simulink model "Test_inverse_kinematics"  (R2017a)
settings: Solver=VariableStepAuto  StartTime=0.0  StopTime=T  RelTol=1e-3
InitFcn:
  | KUKA_LBR_init
values from neighbouring files (symbols this model uses):
  elbowAngle = elbowAngle * pi/180    (= 0)    [KUKA_LBR_init.m]    (also in Untitled2.m)
  Kuka_LBR_param_simu = Simulink.Parameter(Kuka_LBR_param_simu)    [KUKA_LBR_init.m]
  rpyDes = rpyDes * pi/180    [KUKA_LBR_init.m]    (also in Untitled2.m)
  T = 0.5    [KUKA_LBR_init.m]
  vecGlobalConfig = [1; 1; 1]    [KUKA_LBR_init.m]    (also in Untitled2.m = [1, 1, 1])
settings Model: Creator=pc  LastModifiedBy=pc

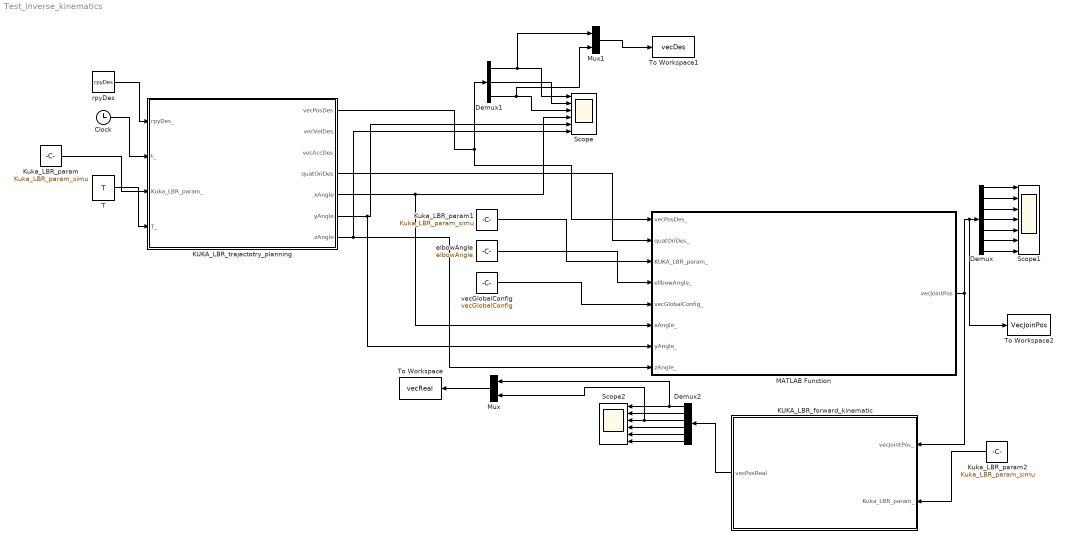
== system Test_inverse_kinematics ==
  Clock : Clock
  Demux : Demux  Outputs=7
  Demux1 : Demux  Outputs=3
  Demux2 : Demux  Outputs=6
  KUKA_LBR_forward_kinematic : MATLAB Function  TreatAsAtomicUnit=on
  KUKA_LBR_trajectotry_planning : MATLAB Function  TreatAsAtomicUnit=on
  Kuka_LBR_param : Constant  Value=Kuka_LBR_param_simu  OutDataTypeStr=Bus: Kuka_LBR_param_simu_Type
  Kuka_LBR_param1 : Constant  Value=Kuka_LBR_param_simu  OutDataTypeStr=Bus: Kuka_LBR_param_simu_Type
  Kuka_LBR_param2 : Constant  Value=Kuka_LBR_param_simu  OutDataTypeStr=Bus: Kuka_LBR_param_simu_Type
  MATLAB Function : MATLAB Function  TreatAsAtomicUnit=on
  Mux : Mux  Inputs=2
  Mux1 : Mux  Inputs=2
  Scope : Scope  NumInputPorts=6
  Scope1 : Scope  NumInputPorts=7
  Scope2 : Scope  NumInputPorts=6
  T : Constant  Value=T
  To Workspace : ToWorkspace  VariableName=vecReal  SaveFormat=Timeseries  SampleTime=-1
  To Workspace1 : ToWorkspace  VariableName=vecDes  SaveFormat=Timeseries  SampleTime=-1
  To Workspace2 : ToWorkspace  VariableName=VecJoinPos  SaveFormat=Timeseries  SampleTime=-1
  elbowAngle : Constant  Value=elbowAngle
  rpyDes : Constant  Value=rpyDes
  vecGlobalConfig : Constant  Value=vecGlobalConfig
  wires:
  Kuka_LBR_param1/1 -> MATLAB Function/3(KUKA_LBR_param_)
  rpyDes/1 -> KUKA_LBR_trajectotry_planning/1(rpyDes_)
  Clock/1 -> KUKA_LBR_trajectotry_planning/2(t_)
  Kuka_LBR_param/1 -> KUKA_LBR_trajectotry_planning/3(Kuka_LBR_param_)
  KUKA_LBR_trajectotry_planning/4(quatOriDes) -> MATLAB Function/2(quatOriDes_)
  T/1 -> KUKA_LBR_trajectotry_planning/4(T_)
  KUKA_LBR_trajectotry_planning/1(vecPosDes) -> Demux1/1, MATLAB Function/1(vecPosDes_)
  vecGlobalConfig/1 -> MATLAB Function/5(vecGlobalConfig_)
  elbowAngle/1 -> MATLAB Function/4(ellbowAngle_)
  MATLAB Function/1(vecJointPos) -> To Workspace2/1, Demux/1, KUKA_LBR_forward_kinematic/1(vecJointPos_)
  Demux/7 -> Scope1/7
  Demux/6 -> Scope1/6
  Demux/5 -> Scope1/5
  Demux/4 -> Scope1/4
  Demux/3 -> Scope1/3
  Demux/2 -> Scope1/2
  Demux/1 -> Scope1/1
  Demux1/1 -> Mux1/1, Scope/1
  Demux1/2 -> Scope/2
  Demux1/3 -> Mux1/2, Scope/3
  Demux2/3 -> Mux/2, Scope2/3
  Demux2/2 -> Scope2/2
  Demux2/1 -> Mux/1, Scope2/1
  KUKA_LBR_forward_kinematic/1(vecPosReal) -> Demux2/1
  Demux2/4 -> Scope2/4
  Demux2/5 -> Scope2/5
  Demux2/6 -> Scope2/6
  Kuka_LBR_param2/1 -> KUKA_LBR_forward_kinematic/2(Kuka_LBR_param_)
  KUKA_LBR_trajectotry_planning/5(xAngle) -> MATLAB Function/6(xAngle_), Scope/4
  KUKA_LBR_trajectotry_planning/6(yAngle) -> MATLAB Function/7(yAngle_), Scope/5
  KUKA_LBR_trajectotry_planning/7(zAngle) -> MATLAB Function/8(zAngle_), Scope/6
  Mux/1 -> To Workspace/1
  Mux1/1 -> To Workspace1/1

== matlab function Test_inverse_kinematics/MATLAB Function ==
  data: vecPosDes_ input; vecJointPos output; quatOriDes_ input; KUKA_LBR_param_ input; ellbowAngle_ input; vecGlobalConfig_ input; xAngle_ input; yAngle_ input; zAngle_ input
function vecJointPos  = KUKA_LBR_iiwa_inverse_kinematic(vecPosDes_,quatOriDes_,KUKA_LBR_param_,ellbowAngle_,vecGlobalConfig_, xAngle_, yAngle_, zAngle_)

 
%  * Creation of a new function that calculates the jointAngles of the robot arm
%  * The function works with three variables which are necessary for calculation
%  * vecJointPos describes the current state of the jointAngles
%  * vecPosDes describes the desired state of the jointAngles
%  quatOriDes describes the desired orientation of the tool as a quaternion
%  

% set Global configuration parameters
if vecGlobalConfig_(1,1) > 0 
    lefty = 1;
else 
    lefty = -1;
end

if vecGlobalConfig_(2,1) > 0 
    ellbowUp = 1;
else 
    ellbowUp = -1;
end

if vecGlobalConfig_(3,1) > 0 
    wristIn = 1;
else 
    wristIn = -1;
end


vecJointPos = [1,1,1,1,1,1,1];

qw = quatOriDes_(1);
qx = quatOriDes_(2);
qy = quatOriDes_(3);
qz = quatOriDes_(4);



rotMatDes = [1-2*qy^2-2*qz^2, 2*qx*qy-2*qz*qw, 2*qx*qz+2*qy*qw; ...
             2*qx*qy+2*qz*qw, 1-2*qx^2-2*qz^2, 2*qy*qz-2*qx*qw; ...
             2*qx*qz-2*qy*qw, 2*qy*qz+2*qx*qw, 1-2*qx^2-2*qy^2];
         

%rotMatDes = rotz(zAngle_)* roty(yAngle_)*rotx(xAngle_);

limitsUpper = zeros(7,1);
limitsLower = zeros(7,1);

% Setting upper and lower limits for different joints
limitsUpper(1,1) = KUKA_LBR_param_.dblJoint1PosMax;
limitsUpper(2,1) = KUKA_LBR_param_.dblJoint2PosMax;
limitsUpper(3,1) = KUKA_LBR_param_.dblJoint3PosMax;
limitsUpper(4,1) = KUKA_LBR_param_.dblJoint4PosMax;
limitsUpper(5,1) = KUKA_LBR_param_.dblJoint5PosMax;
limitsUpper(6,1) = KUKA_LBR_param_.dblJoint6PosMax;
limitsUpper(7,1) = KUKA_LBR_param_.dblJoint7PosMax;

limitsLower(1,1) = KUKA_LBR_param_.dblJoint1PosMin;
limitsLower(2,1) = KUKA_LBR_param_.dblJoint2PosMin;
limitsLower(3,1) = KUKA_LBR_param_.dblJoint3PosMin;
limitsLower(4,1) = KUKA_LBR_param_.dblJoint4PosMin;
limitsLower(5,1) = KUKA_LBR_param_.dblJoint5PosMin;
limitsLower(6,1) = KUKA_LBR_param_.dblJoint6PosMin;
limitsLower(7,1) = KUKA_LBR_param_.dblJoint7PosMin;

%Vector from Base to shoulder
vecBasetoJoint2 = [0,0,KUKA_LBR_param_.dblLinkBase1Len]';

%Vector from Wrist to endeffector
vecJoint6to7 = [0,0,KUKA_LBR_param_.dblLink67Len]';

%vector from shoulder to wrist

vecJoint2to6 = vecPosDes_' - vecBasetoJoint2 - (rotMatDes * vecJoint6to7);

%calculate unit vector from shoulder to wrist

distJoint2To6 = norm(vecJoint2to6);

vecDirectionJoint2To6 = vecJoint2to6/distJoint2To6;

skewMatDirJoint2to6 = zeros(3,3);

skewMatDirJoint2to6(1,1) = 0;
skewMatDirJoint2to6(1,2) = -vecDirectionJoint2To6(3,1);
skewMatDirJoint2to6(1,3) = vecDirectionJoint2To6(2,1);
skewMatDirJoint2to6(2,1) = vecDirectionJoint2To6(3,1);
skewMatDirJoint2to6(2,2) = 0;
skewMatDirJoint2to6(2,3) = -vecDirectionJoint2To6(1,1);
skewMatDirJoint2to6(3,1) = -vecDirectionJoint2To6(2,1);
skewMatDirJoint2to6(3,2) = vecDirectionJoint2To6(1,1);
skewMatDirJoint2to6(3,3) = 0;

argument4 = (distJoint2To6.^2 - KUKA_LBR_param_.dblLink23Len.^2 - KUKA_LBR_param_.dblLink45Len.^2)/(2 * KUKA_LBR_param_.dblLink45Len *  KUKA_LBR_param_.dblLink23Len);

referenceAngle4 = ellbowUp * real(acos(checkArgument(argument4)));

if (referenceAngle4 > limitsUpper(4,1) || referenceAngle4 < limitsLower(4,1) || isnan(referenceAngle4))
    error('limits of joint Angle 4 exceeded');
        

end

%calculation of help angles alpha and beta

argument_alpha = vecJoint2to6(3,1) / distJoint2To6;

alpha = asin(checkArgument(argument_alpha));

argument_beta = (KUKA_LBR_param_.dblLink23Len.^2 + distJoint2To6.^2 - KUKA_LBR_param_.dblLink45Len.^2)/( 2 * KUKA_LBR_param_.dblLink23Len * distJoint2To6);

beta = acos(checkArgument(argument_beta));

%calculation of reference Angle 1 wih alpha and beta

referenceAngle1 = atan2(vecJoint2to6(2,1),vecJoint2to6(1,1));

referenceAngle2 = pi/2 - alpha - ellbowUp * beta;

referenceAngle3 = 0;

%vecReferenceAngles = [referenceAngle1 , referenceAngle2, referenceAngle3, referenceAngle4];

IMat3x3 = eye(3);

rotMatEllbowAngle = IMat3x3 + sin(ellbowAngle_) * skewMatDirJoint2to6 + (1-cos(ellbowAngle_)) * skewMatDirJoint2to6.^2;

veclinklengths = [KUKA_LBR_param_.dblLinkBase1Len; 0; KUKA_LBR_param_.dblLink23Len; 0; KUKA_LBR_param_.dblLink45Len; 0; KUKA_LBR_param_.dblLink67Len];

vecRotbetweenJoints = [-pi/2, pi/2,pi/2,-pi/2,-pi/2,pi/2,0];

refTransMat0to1 = denavitHardenbergTransformation(vecRotbetweenJoints(1,1), referenceAngle1, veclinklengths(1));

refTransMat1to2 = denavitHardenbergTransformation(vecRotbetweenJoints(1,2), referenceAngle2, veclinklengths(2));

refTransMat2to3 = denavitHardenbergTransformation(vecRotbetweenJoints(1,3), referenceAngle3, veclinklengths(3));

refTransMat3to4 = denavitHardenbergTransformation(vecRotbetweenJoints(1,4), referenceAngle4, veclinklengths(4));

refTransMat0to3 = refTransMat0to1 * refTransMat1to2 * refTransMat2to3;

refTransMat0to4 = refTransMat0to3 * refTransMat3to4;


%Identification of the rotation matrices of the refernce syste%

refRotMat0to3 = refTransMat0to3(1:3,1:3);

refRotMat0to4 = refTransMat0to4(1:3,1:3);

coeffMatAs = skewMatDirJoint2to6 * refRotMat0to3;

coeffMatBs = - (skewMatDirJoint2to6 * skewMatDirJoint2to6) * refRotMat0to3;

coeffMatCs = (vecDirectionJoint2To6 *vecDirectionJoint2To6' ) * refRotMat0to3;

argument1Nominator = -coeffMatAs(2,2) * sin(ellbowAngle_) ...
         - coeffMatBs(2,2) * cos(ellbowAngle_) - coeffMatCs(2,2);
     
     if argument1Nominator < 1e-4 && argument1Nominator > -1e-4
        jointAngle1 = 0;
     else
        jointAngle1 = atan2(lefty * (-coeffMatAs(2,2) * sin(ellbowAngle_) ...
         - coeffMatBs(2,2) * cos(ellbowAngle_) - coeffMatCs(2,2)), ...
          lefty * (coeffMatAs(1,2) * sin(ellbowAngle_) ... 
          - coeffMatBs(1,2) * cos(ellbowAngle_) - coeffMatCs(1,2)));
     end  
if (jointAngle1 > limitsUpper(1,1) || jointAngle1 < limitsLower(1,1)) 
    error('Limits of joinAngle1 exceeded!');
        
end

argument2 = coeffMatAs(3,2) * sin(ellbowAngle_) ...
             + coeffMatBs(3,2) * cos(ellbowAngle_) ...
             + coeffMatCs(3,2);
        
jointAngle2 = lefty * acos(checkArgument(argument2));

if (jointAngle2 > limitsUpper(2,1) || jointAngle2 < limitsLower(2,1))
    error('Limits of joinAngle2 exceeded!');
        
end

argument3Nominator = -lefty * (coeffMatAs(3,3) * sin(ellbowAngle_) ...
                    + coeffMatBs(3,3) * cos(ellbowAngle_) ...
                     + coeffMatCs(3,3));
                 
if argument3Nominator < 1e-4 && argument3Nominator > -1e-4
    jointAngle3 = 0;
    
else
jointAngle3 = atan2(-lefty * (coeffMatAs(3,3) * sin(ellbowAngle_) ...
                    + coeffMatBs(3,3) * cos(ellbowAngle_) ...
                     + coeffMatCs(3,3)), ... 
                    lefty * (-coeffMatAs(3,1) * sin(ellbowAngle_)...
                    - coeffMatBs(3,1) * cos(ellbowAngle_) ...
                    - coeffMatCs(3,1)));
end

if (jointAngle3 > limitsUpper(3,1) || jointAngle3 < limitsLower(3,1))
   error('Limits of joinAngle3 exceeded!');
        
end

jointAngle4 = referenceAngle4;

if (jointAngle4 > limitsUpper(4,1) || jointAngle4 < limitsLower(4,1))
    error('Limits of joinAngle4 exceeded!');
      
end

rotMat0to3 = rotMatEllbowAngle * refRotMat0to3;
rotMat0to4 = rotMatEllbowAngle * refRotMat0to4;
rotMat3to4 = transpose(rotMat0to3) * rotMat0to4;

coeffMatAw = transpose(rotMat3to4) * transpose(coeffMatAs) * rotMatDes;
coeffMatBw = transpose(rotMat3to4) * transpose(coeffMatBs) * rotMatDes;
coeffMatCw = transpose(rotMat3to4) * transpose(coeffMatCs) * rotMatDes;


%Calculation of jointAngle5 with the coefficient matrices
argument5Nominator = wristIn * coeffMatAw(2,3) * sin(ellbowAngle_) ...
              + coeffMatBw(2,3) * cos(ellbowAngle_) ... 
              + coeffMatCw(2,3);
                 
if argument5Nominator < 1e-4 && argument5Nominator > -1e-4
    jointAngle5 = 0;
    
else
    
jointAngle5 = atan2(wristIn * coeffMatAw(2,3) * sin(ellbowAngle_) ...
              + coeffMatBw(2,3) * cos(ellbowAngle_) ... 
              + coeffMatCw(2,3), ...
              wristIn *(coeffMatAw(1,3) * sin(ellbowAngle_) ...
              + coeffMatBw(1,3) * cos(ellbowAngle_) ...
              + coeffMatCw(1,3)));

end
if (jointAngle5 > limitsUpper(5,1) || jointAngle5 < limitsLower(5,1))
     error('Limits of joinAngle5 exceeded!');
      
end 


    
argument6 = coeffMatAw(3,3) * sin(ellbowAngle_) ...
            + coeffMatBw(3,3) * cos(ellbowAngle_) ...
                  + coeffMatCw(3,3);

jointAngle6 = wristIn * acos(checkArgument(argument6));

if (jointAngle6 > limitsUpper(6,1) || jointAngle6 < limitsLower(6,1))
      error('Limits of joinAngle6 exceeded!');
      
end 

argument7Nominator = wristIn * (coeffMatAw(3,2) * sin(ellbowAngle_) ...
            + coeffMatBw(3,2) * cos(ellbowAngle_) ...
            + coeffMatCw(3,2));
                 
if argument7Nominator < 1e-4 && argument7Nominator > -1e-4
    jointAngle7 = 0;    
else
jointAngle7 = atan2(wristIn * (coeffMatAw(3,2) * sin(ellbowAngle_) ...
            + coeffMatBw(3,2) * cos(ellbowAngle_) ...
            + coeffMatCw(3,2)), ...
            wristIn * (-coeffMatAw(3,1) * sin(ellbowAngle_) ...
            - coeffMatBw(3,1) * cos(ellbowAngle_)...
            -coeffMatCw(3,1)));
end

if (jointAngle7 > limitsUpper(7,1) || jointAngle7 < limitsLower(7,1))
       error('Limits of joinAngle7 exceeded!');
        
end

    vecJointPos(1) = jointAngle1;
    vecJointPos(2) = jointAngle2;
    vecJointPos(3) = jointAngle3;
    vecJointPos(4) = -jointAngle4;
    vecJointPos(5) = jointAngle5;
    vecJointPos(6) = jointAngle6;
    vecJointPos(7) = jointAngle7;
end



function [rotmat] = denavitHardenbergTransformation(alpha_,theta_,d_)


matRot = rotz(theta_) *rotx(alpha_);

vecTrans = [0;0;d_];

matTrans = [matRot vecTrans];

rotmat = [matTrans; 0 0 0 1];

end

function [argument_] = checkArgument(argument_)

if argument_ < -1.0
    if argument_ < -1.001
        error('Invalid Argument');
        
    else
        argument_ = -1.0;
    end
elseif argument_ > 1.0
        if argument_ > 1.001
            error('Invalid Argument');
        
        
    else
        argument_ = 1.0;
        end
end
end


function rotxAlpha  = rotx(alpha_)
rotxAlpha = [1 0           0; ...
             0 cos(alpha_) -sin(alpha_); ... 
             0 sin(alpha_) cos(alpha_)];
end

function rotzTheta  = rotz(theta_)
rotzTheta = [cos(theta_) -sin(theta_) 0; ... 
             sin(theta_) cos(theta_)  0; ...
             0           0            1];
end

function roty = roty(theta_)
roty = [     cos(theta_)  0   sin(theta_) ; ... 
             0            1   0             ; ...
             -sin(theta_)  0   cos(theta_)];
end

== matlab function Test_inverse_kinematics/KUKA_LBR_forward_kinematic ==
  data: vecJointPos_ input; vecPosReal output; Kuka_LBR_param_ input
function vecPosReal = KUKA_LBR_forward_kinematic(vecJointPos_,Kuka_LBR_param_)

q1 = vecJointPos_(1);
q2 = vecJointPos_(2);
q3 = vecJointPos_(3);
q4 = vecJointPos_(4);
q5 = vecJointPos_(5);
q6 = vecJointPos_(6);
q7 = vecJointPos_(7);

T07 = [cos(q7).*(cos(q6).*(cos(q5).*(cos(q4).*(cos(q1).*cos(q2).*cos(q3)+(-1) ...
  .*sin(q1).*sin(q3))+cos(q1).*sin(q2).*sin(q4))+((-1).*cos(q3).*sin(q1)+( ...
  -1).*cos(q1).*cos(q2).*sin(q3)).*sin(q5))+((-1).*cos(q1).*cos(q4).*sin( ...
  q2)+(cos(q1).*cos(q2).*cos(q3)+(-1).*sin(q1).*sin(q3)).*sin(q4)).*sin( ...
  q6))+(cos(q5).*((-1).*cos(q3).*sin(q1)+(-1).*cos(q1).*cos(q2).*sin(q3))+ ...
  (-1).*(cos(q4).*(cos(q1).*cos(q2).*cos(q3)+(-1).*sin(q1).*sin(q3))+cos( ...
  q1).*sin(q2).*sin(q4)).*sin(q5)).*sin(q7),cos(q7).*(cos(q5).*((-1).*cos( ...
  q3).*sin(q1)+(-1).*cos(q1).*cos(q2).*sin(q3))+(-1).*(cos(q4).*(cos(q1).* ...
  cos(q2).*cos(q3)+(-1).*sin(q1).*sin(q3))+cos(q1).*sin(q2).*sin(q4)).* ...
  sin(q5))+(-1).*(cos(q6).*(cos(q5).*(cos(q4).*(cos(q1).*cos(q2).*cos(q3)+ ...
  (-1).*sin(q1).*sin(q3))+cos(q1).*sin(q2).*sin(q4))+((-1).*cos(q3).*sin( ...
  q1)+(-1).*cos(q1).*cos(q2).*sin(q3)).*sin(q5))+((-1).*cos(q1).*cos(q4).* ...
  sin(q2)+(cos(q1).*cos(q2).*cos(q3)+(-1).*sin(q1).*sin(q3)).*sin(q4)).* ...
  sin(q6)).*sin(q7),(-1).*cos(q6).*((-1).*cos(q1).*cos(q4).*sin(q2)+(cos( ...
  q1).*cos(q2).*cos(q3)+(-1).*sin(q1).*sin(q3)).*sin(q4))+(cos(q5).*(cos( ...
  q4).*(cos(q1).*cos(q2).*cos(q3)+(-1).*sin(q1).*sin(q3))+cos(q1).*sin(q2) ...
  .*sin(q4))+((-1).*cos(q3).*sin(q1)+(-1).*cos(q1).*cos(q2).*sin(q3)).* ...
  sin(q5)).*sin(q6),Kuka_LBR_param_.dblLink23Len.*cos(q1).*sin(q2)+Kuka_LBR_param_.dblLink45Len.*(cos(q1).*cos(q4).*sin(q2)+ ...
  (-1).*(cos(q1).*cos(q2).*cos(q3)+(-1).*sin(q1).*sin(q3)).*sin(q4))+Kuka_LBR_param_.dblLink67Len.* ...
  ((-1).*cos(q6).*((-1).*cos(q1).*cos(q4).*sin(q2)+(cos(q1).*cos(q2).*cos( ...
  q3)+(-1).*sin(q1).*sin(q3)).*sin(q4))+(cos(q5).*(cos(q4).*(cos(q1).*cos( ...
  q2).*cos(q3)+(-1).*sin(q1).*sin(q3))+cos(q1).*sin(q2).*sin(q4))+((-1).* ...
  cos(q3).*sin(q1)+(-1).*cos(q1).*cos(q2).*sin(q3)).*sin(q5)).*sin(q6)); ...
  cos(q7).*(cos(q6).*(cos(q5).*(cos(q4).*(cos(q2).*cos(q3).*sin(q1)+cos( ...
  q1).*sin(q3))+sin(q1).*sin(q2).*sin(q4))+(cos(q1).*cos(q3)+(-1).*cos(q2) ...
  .*sin(q1).*sin(q3)).*sin(q5))+((-1).*cos(q4).*sin(q1).*sin(q2)+(cos(q2) ...
  .*cos(q3).*sin(q1)+cos(q1).*sin(q3)).*sin(q4)).*sin(q6))+(cos(q5).*(cos( ...
  q1).*cos(q3)+(-1).*cos(q2).*sin(q1).*sin(q3))+(-1).*(cos(q4).*(cos(q2).* ...
  cos(q3).*sin(q1)+cos(q1).*sin(q3))+sin(q1).*sin(q2).*sin(q4)).*sin(q5)) ...
  .*sin(q7),cos(q7).*(cos(q5).*(cos(q1).*cos(q3)+(-1).*cos(q2).*sin(q1).* ...
  sin(q3))+(-1).*(cos(q4).*(cos(q2).*cos(q3).*sin(q1)+cos(q1).*sin(q3))+ ...
  sin(q1).*sin(q2).*sin(q4)).*sin(q5))+(-1).*(cos(q6).*(cos(q5).*(cos(q4) ...
  .*(cos(q2).*cos(q3).*sin(q1)+cos(q1).*sin(q3))+sin(q1).*sin(q2).*sin(q4) ...
  )+(cos(q1).*cos(q3)+(-1).*cos(q2).*sin(q1).*sin(q3)).*sin(q5))+((-1).* ...
  cos(q4).*sin(q1).*sin(q2)+(cos(q2).*cos(q3).*sin(q1)+cos(q1).*sin(q3)).* ...
  sin(q4)).*sin(q6)).*sin(q7),(-1).*cos(q6).*((-1).*cos(q4).*sin(q1).*sin( ...
  q2)+(cos(q2).*cos(q3).*sin(q1)+cos(q1).*sin(q3)).*sin(q4))+(cos(q5).*( ...
  cos(q4).*(cos(q2).*cos(q3).*sin(q1)+cos(q1).*sin(q3))+sin(q1).*sin(q2).* ...
  sin(q4))+(cos(q1).*cos(q3)+(-1).*cos(q2).*sin(q1).*sin(q3)).*sin(q5)).* ...
  sin(q6),Kuka_LBR_param_.dblLink23Len.*sin(q1).*sin(q2)+Kuka_LBR_param_.dblLink45Len.*(cos(q4).*sin(q1).*sin(q2)+(-1).*( ...
  cos(q2).*cos(q3).*sin(q1)+cos(q1).*sin(q3)).*sin(q4))+Kuka_LBR_param_.dblLink67Len.*((-1).*cos( ...
  q6).*((-1).*cos(q4).*sin(q1).*sin(q2)+(cos(q2).*cos(q3).*sin(q1)+cos(q1) ...
  .*sin(q3)).*sin(q4))+(cos(q5).*(cos(q4).*(cos(q2).*cos(q3).*sin(q1)+cos( ...
  q1).*sin(q3))+sin(q1).*sin(q2).*sin(q4))+(cos(q1).*cos(q3)+(-1).*cos(q2) ...
  .*sin(q1).*sin(q3)).*sin(q5)).*sin(q6));cos(q7).*(cos(q6).*(cos(q5).*(( ...
  -1).*cos(q3).*cos(q4).*sin(q2)+cos(q2).*sin(q4))+sin(q2).*sin(q3).*sin( ...
  q5))+((-1).*cos(q2).*cos(q4)+(-1).*cos(q3).*sin(q2).*sin(q4)).*sin(q6))+ ...
  (cos(q5).*sin(q2).*sin(q3)+(-1).*((-1).*cos(q3).*cos(q4).*sin(q2)+cos( ...
  q2).*sin(q4)).*sin(q5)).*sin(q7),cos(q7).*(cos(q5).*sin(q2).*sin(q3)+( ...
  -1).*((-1).*cos(q3).*cos(q4).*sin(q2)+cos(q2).*sin(q4)).*sin(q5))+(-1).* ...
  (cos(q6).*(cos(q5).*((-1).*cos(q3).*cos(q4).*sin(q2)+cos(q2).*sin(q4))+ ...
  sin(q2).*sin(q3).*sin(q5))+((-1).*cos(q2).*cos(q4)+(-1).*cos(q3).*sin( ...
  q2).*sin(q4)).*sin(q6)).*sin(q7),(-1).*cos(q6).*((-1).*cos(q2).*cos(q4)+ ...
  (-1).*cos(q3).*sin(q2).*sin(q4))+(cos(q5).*((-1).*cos(q3).*cos(q4).*sin( ...
  q2)+cos(q2).*sin(q4))+sin(q2).*sin(q3).*sin(q5)).*sin(q6),Kuka_LBR_param_.dblLinkBase1Len + Kuka_LBR_param_.dblLink23Len.*cos(q2)+ ...
  Kuka_LBR_param_.dblLink45Len.*(cos(q2).*cos(q4)+cos(q3).*sin(q2).*sin(q4))+Kuka_LBR_param_.dblLink67Len.*((-1).*cos(q6).*( ...
  (-1).*cos(q2).*cos(q4)+(-1).*cos(q3).*sin(q2).*sin(q4))+(cos(q5).*((-1) ...
  .*cos(q3).*cos(q4).*sin(q2)+cos(q2).*sin(q4))+sin(q2).*sin(q3).*sin(q5)) ...
  .*sin(q6));0,0,0,1];

phibe = atan(T07(2,1)/T07(1,1));
thetabe = atan(T07(3,1)/sqrt(T07(3,2).^2+T07(3,3).^2));
psibe = atan(T07(3,2)/T07(3,3));

xdblTool = [Kuka_LBR_param_.dblToolLenX; Kuka_LBR_param_.dblToolLenY; Kuka_LBR_param_.dblToolLenZ; 1];
xbe      = T07*[0;0;0;1];

vecPosReal = [xbe(1); xbe(2); xbe(3); phibe; thetabe; psibe]';

== matlab function Test_inverse_kinematics/KUKA_LBR_trajectotry_planning ==
  data: vecPosDes output; vecVelDes output; vecAccDes output; rpyDes_ input; quatOriDes output; t_ input; Kuka_LBR_param_ input; T_ input; xAngle output; yAngle output; zAngle output
function [vecPosDes, vecVelDes, vecAccDes, quatOriDes, xAngle, yAngle, zAngle] = KUKA_LBR_trajectotry_planning(rpyDes_, t_, Kuka_LBR_param_,T_)
%Abbreviations for the various angular function

    xAngle = rpyDes_(1);
    yAngle = -pi/5*t_; %rpyDes_(2);
    zAngle = rpyDes_(3);
    

    cy = cos(zAngle * 0.5);
    sy = sin(zAngle * 0.5);
    cp = cos(yAngle * 0.5);
    sp = sin(yAngle * 0.5);
    cr = cos(xAngle * 0.5);
    sr = sin(xAngle * 0.5);

    q = [1 1 1 1];
    q(1) = cy * cp * cr + sy * sp * sr;
    q(2) = cy * cp * sr - sy * sp * cr;
    q(3) = sy * cp * sr + cy * sp * cr;
    q(4) = sy * cp * cr - cy * sp * sr;
    
    KUKA_length = Kuka_LBR_param_.dblLinkBase1Len + Kuka_LBR_param_.dblLink23Len + ...
                  Kuka_LBR_param_.dblLink45Len +  Kuka_LBR_param_.dblLink67Len; 
              
    xe= Kuka_LBR_param_.dblLink23Len + Kuka_LBR_param_.dblLink45Len +  Kuka_LBR_param_.dblLink67Len; 
    
    x = t_*xe;
    y = 0;
    z = t_*Kuka_LBR_param_.dblLinkBase1Len + (1-t_)*KUKA_length ;
    
    x_dot = xe;
    y_dot = 0;
    z_dot = - 1/3 * KUKA_length;

%     x = KUKA_length/(3*sin(pi/6)*T_) * t_ * 0;
%     y = 0;
%     z = KUKA_length - (KUKA_length/3*T_) * t_ * 0;
%     
%     x_dot = (2*KUKA_length) / (3*T_) * 0;
%     y_dot = 0;
%     z_dot = - KUKA_length / (3*T_) * 0;

    
    x_ddot = 0;
    y_ddot = 0;
    z_ddot = 0;
    
vecPosDes  = [x y z];    
vecVelDes  = [x_dot y_dot z_dot];
vecAccDes  = [x_ddot y_ddot z_ddot];
quatOriDes = q;
